simulink model "mbd_example_led"  (R2022b)
settings: Solver=FixedStepDiscrete  StartTime=0.0  StopTime=10.0  RelTol=1e-3  EnableMultiTasking=on
PostLoadFcn:
  | run([bdroot '_init']);
InitFcn:
  | checkModelFolder(true); % Optional
  | run([bdroot '_init']);
values from neighbouring files (symbols this model uses):
  T_s_LED1 = 1/LED1_Hz    (= 0.5)    [mbd_example_led_init.m]
  T_s_LED2 = 1/LED2_Hz    (= 1)    [mbd_example_led_init.m]
libraries: MbdLib_Digital x15, MbdLib_Timer x7, MbdLib_Sys x4, MbdLib_Required x1
(part 2 of 2)

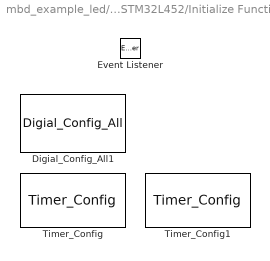
== system mbd_example_led/Variant Subsystem/STM32L452/Initialize Function ==
  Digial_Config_All1 : MbdLib_Digital/Digial_Config_All  Priority=30  Param_channels={ 'A', '0', 'off', '0 : input', '0 : low', '0 : none', '0 : none', '0 : low', '0 : low'; 'A', '1', 'off', '0 : input', '0 : low', '0 : none', '0 : none', '0 : low', '0 : low'; 'A', '2', 'off', '0 : input', '0 : low', '0 : none', '0 : none', '0 : low', '0 : low'; 'A', '3', 'off', '0 : input', '0 : low', '0 : none', '0 : none', '0 : low', '0 : low'; 'A', '4', 'off', '0 : input', '0 : low', '0 : none', '0 : none', '0 : low', '0 : low'; 'A', '5', 'off', '0 : input', '0 : low', '0 : none', '0 : none', '0 : low', '0 : low'; 'A', '6', 'off', '0 : input', '0 : low', '0 : none', '0 : none', '0 : low', '0 : low'; 'A', '7', 'off', '0 : input', '0 : low', '0 : none', '0 : none', '0 : low', '0 : low'; 'A', '8', 'off', '0 : input', '0 : low', '0 : none', '0 : none', '0 : low', '0 : low'; 'A', '9', 'off', '0 : input', '0 : low', '0 : none', '0 : none', '0 : low', '0 : low'; 'A', '10', 'off', '0 : input', '0 : low', '0 : none', '0 : none', '0 : low', '0 : low'; 'A', '11', 'off', '0 : input', '0 : low', '0 : none', '0 : none', '0 : low', '0 : low'; 'A', '12', 'off', '0 : input', '0 : low', '0 : none', '0 : none', '0 : low', '0 : low'; 'A', '13', 'off', '0 : input', '0 : low', '0 : none', '0 : none', '0 : low', '0 : low'; 'A', '14', 'off', '0 : input', '0 : low', '0 : none', '0 : none', '0 : low', '0 : low'; 'A', '15', 'off', '0 : input', '0 : low', '0 : none', '0 : none', '0 : low', '0 : low'; 'A', '16', 'off', '0 : input', '0 : low', '0 : none', '0 : none', '0 : low', '0 : low'; 'A', '17', 'off', '0 : input', '0 : low', '0 : none', '0 : none', '0 : low', '0 : low'; 'A', '18', 'off', '0 : input', '0 : low', '0 : none', '0 : none', '0 : low', '0 : low'; 'A', '19', 'off', '0 : input', '0 : low', '0 : none', '0 : none', '0 : low', '0 : low'; 'A', '20', 'off', '0 : input', '0 : low', '0 : none', '0 : none', '0 : low', '0 : low'; 'A', '21', 'off', '0 : input', '0 : low', '0 : none', '0 : none', '0 : low', '0 : low'; 'A', '22', 'off', '0 : input', '0 : low', '0 : none', '0 : none', '0 : low', '0 : low'; 'A', '23', 'off', '0 : input', '0 : low', '0 : none', '0 : none', '0 : low', '0 : low'; 'A', '24', 'off', '0 : input', '0 : low', '0 : none', '0 : none', '0 : low', '0 : low'; 'A', '25', 'off', '0 : input', '0 : low', '0 : none', '0 : none', '0 : low', '0 : low'; 'A', '26', 'off', '0 : input', '0 : low', '0 : none', '0 : none', '0 : low', '0 : low'; 'A', '27', 'off', '0 : input', '0 : low', '0 : none', '0 : none', '0 : low', '0 : low'; 'A', '28', 'off', '0 : input', '0 : low', '0 : none', '0 : none', '0 : low', '0 : low'; 'A', '29', 'off', '0 : input', '0 : low', '0 : none', '0 : none', '0 : low', '0 : low'; 'A', '30', 'off', '0 : input', '0 : low', '0 : none', '0 : none', '0 : low', '0 : low'; 'A', '31', 'off', '0 : input', '0 : low', '0 : none', '0 : none', '0 : low', '0 : low'; 'B', '0', 'off', '0 : input', '0 : low', '0 : none', '0 : none', '0 : low', '0 : low'; 'B', '1', 'off', '0 : input', '0 : low', '0 : none', '0 : none', '0 : low', '0 : low'; 'B', '2', 'off', '0 : input', '0 : low', '0 : none', '0 : none', '0 : low', '0 : low'; 'B', '3', 'off', '0 : input', '0 : low', '0 : none', '0 : none', '0 : low', '0 : low'; 'B', '4', 'off', '0 : input', '0 : low', '0 : none', '0 : none', '0 : low', '0 : low'; 'B', '5', 'off', '0 : input', '0 : low', '0 : none', '0 : none', '0 : low', '0 : low'; 'B', '6', 'off', '0 : input', '0 : low', '0 : none', '0 : none', '0 : low', '0 : low'; 'B', '7', 'off', '0 : input', '0 : low', '0 : none', '0 : none', '0 : low', '0 : low'; 'B', '8', 'off', '0 : input', '0 : low', '0 : none', '0 : none', '0 : low', '0 : low'; 'B', '9', 'off', '0 : input', '0 : low', '0 : none', '0 : none', '0 : low', '0 : low'; 'B', '10', 'off', '0 : input', '0 : low', '0 : none', '0 : none', '0 : low', '0 : low'; 'B', '11', 'off', '0 : input', '0 : low', '0 : none', '0 : none', '0 : low', '0 : low'; 'B', '12', 'off', '0 : input', '0 : low', '0 : none', '0 : none', '0 : low', '0 : low'; 'B', '13', 'off', '0 : input', '0 : low', '0 : none', '0 : none', '0 : low', '0 : low'; 'C', '0', 'off', '0 : input', '0 : low', '0 : none', '0 : none', '0 : low', '0 : low'; 'C', '1', 'off', '0 : input', '0 : low', '0 : none', '0 : none', '0 : low', '0 : low'; 'C', '2', 'off', '0 : input', '0 : low', '0 : none', '0 : none', '0 : low', '0 : low'; 'C', '3', 'off', '0 : input', '0 : low', '0 : none', '0 : none', '0 : low', '0 : low'; 'C', '4', 'off', '0 : input', '0 : low', '0 : none', '0 : none', '0 : low', '0 : low'; 'C', '5', 'off', '0 : input', '0 : low', '0 : none', '0 : none', '0 : low', '0 : low'; 'C', '6', 'off', '0 : input', '0 : low', '0 : none', '0 : none', '0 : low', '0 : low'; 'C', '7', 'off', '0 : input', '0 : low', '0 : none', '0 : none', '0 : low', '0 : low'; 'C', '8', 'off', '0 : input', '0 : low', '0 : none', '0 : none', '0 : low', '0 : low'; 'C', '9', 'off', '0 : input', '0 : low', '0 : none', '0 : none', '0 : low', '0 : low'; 'C', '10', 'on', '1 : output', '0 : low', '0 : none', '0 : none', '0 : low', '0 : low'; 'C', '11', 'off', '0 : input', '0 : low', '0 : none', '0 : none', '0 : low', '0 : low'; 'C', '12', 'off', '0 : input', '0 : low', '0 : none', '0 : none', '0 : low', '0 : low'; 'C', '13', 'on', '0 : input', '0 : low', '0 : none', '1 : pullup', '0 : low', '0 : low'; 'C', '14', 'off', '0 : input', '0 : low', '0 : none', '0 : none', '0 : low', '0 : low'; 'C', '15', 'off', '0 : input', '0 : low', '0 : none', '0 : none', '0 : low', '0 : low'; 'C', '16', 'off', '0 : input', '0 : low', '0 : none', '0 : none', '0 : low', '0 : low'; 'C', '17', 'off', '0 : input', '0 : low', '0 : none', '0 : none', '0 : low', '0 : low'; 'C', '18', 'off', '0 : input', '0 : low', '0 : none', '0 : none', '0 : low', '0 : low'; 'C', '19', 'off', '0 : input', '0 : low', '0 : none', '0 : none', '0 : low', '0 : low'; 'C', '20', 'off', '0 : input', '0 : low', '0 : none', '0 : none', '0 : low', '0 : low'; 'C', '21', 'off', '0 : input', '0 : low', '0 : none', '0 : none', '0 : low', '0 : low'; 'C', '22', 'off', '0 : input', '0 : low', '0 : none', '0 : none', '0 : low', '0 : low'; 'C', '23', 'off', '0 : input', '0 : low', '0 : none', '0 : none', '0 : low', '0 : low'; 'C', '24', 'off', '0 : input', '0 : low', '0 : none', '0 : none', '0 : low', '0 : low'; 'C', '25', 'off', '0 : input', '0 : low', '0 : none', '0 : none', '0 : low', '0 : low'; 'C', '26', 'off', '0 : input', '0 : low', '0 : none', '0 : none', '0 : low', '0 : low'; 'C', '27', 'off', '0 : input', '0 : low', '0 : none', '0 : none', '0 : low', '0 : low'; 'C', '28', 'off', '0 : input', '0 : low', '0 : none', '0 : none', '0 : low', '0 : low'; 'C', '29', 'off', '0 : input', '0 : low', '0 : none', '0 : none', '0 : low', '0 : low'; 'C', '30', 'off', '0 : input', '0 : low', '0 : none', '0 : none', '0 : low', '0 : low'; 'C', '31', 'off', '0 : input', '0 : low', '0 : none', '0 : none', '0 : low', '0 : low'; 'D', '0', 'off', '0 : input', '0 : low', '0 : none', '0 : none', '0 : low', '0 : low'; 'D', '1', 'off', '0 : input', '0 : low', '0 : none', '0 : none', '0 : low', '0 : low'; 'D', '2', 'off', '0 : input', '0 : low', '0 : none', '0 : none', '0 : low', '0 : low'; 'D', '3', 'off', '0 : input', '0 : low', '0 : none', '0 : none', '0 : low', '0 : low'; 'D', '4', 'off', '0 : input', '0 : low', '0 : none', '0 : none', '0 : low', '0 : low'; 'D', '5', 'off', '0 : input', '0 : low', '0 : none', '0 : none', '0 : low', '0 : low'; 'D', '6', 'off', '0 : input', '0 : low', '0 : none', '0 : none', '0 : low', '0 : low'; 'D', '7', 'off', '0 : input', '0 : low', '0 : none', '0 : none', '0 : low', '0 : low'; 'D', '8', 'off', '0 : input', '0 : low', '0 : none', '0 : none', '0 : low', '0 : low'; 'D', '9', 'off', '0 : input', '0 : low', '0 : none', '0 : none', '0 : low', '0 : low'; 'D', '10', 'off', '0 : input', '0 : low', '0 : none', '0 : none', '0 : low', '0 : low'; 'D', '11', 'off', '0 : input', '0 : low', '0 : none', '0 : none', '0 : low', '0 : low'; 'D', '12', 'off', '0 : input', '0 : low', '0 : none', '0 : none', '0 : low', '0 : low'; 'D', '13', 'off', '0 : input', '0 : low', '0 : none', '0 : none', '0 : low', '0 : low'; 'D', '14', 'off', '0 : input', '0 : low', '0 : none', '0 : none', '0 : low', '0 : low'; 'D', '15', 'off', '0 : input', '0 : low', '0 : none', '0 : none', '0 : low', '0 : low'; 'D', '16', 'off', '0 : input', '0 : low', '0 : none', '0 : none', '0 : low', '0 : low'; 'D', '17', 'off', '0 : input', '0 : low', '0 : none', '0 : none', '0 : low', '0 : low'; 'D', '18', 'off', '0 : input', '0 : low', '0 : none', '0 : none', '0 : low', '0 : low'; 'D', '19', 'off', '0 : input', '0 : low', '0 : none', '0 : none', '0 : low', '0 : low'; 'D', '20', 'off', '0 : input', '0 : low', '0 : none', '0 : none', '0 : low', '0 : low'; 'D', '21', 'off', '0 : input', '0 : low', '0 : none', '0 : none', '0 : low', '0 : low'; 'D', '22', 'off', '0 : input', '0 : low', '0 : none', '0 : none', '0 : low', '0 : low'; 'D', '23', 'off', '0 : input', '0 : low', '0 : none', '0 : none', '0 : low', '0 : low'; 'D', '24', 'off', '0 : input', '0 : low', '0 : none', '0 : none', '0 : low', '0 : low'; 'D', '25', 'off', '0 : input', '0 : low', '0 : none', '0 : none', '0 : low', '0 : low'; 'D', '26', 'off', '0 : input', '0 : low', '0 : none', '0 : none', '0 : low', '0 : low'; 'D', '27', 'off', '0 : input', '0 : low', '0 : none', '0 : none', '0 : low', '0 : low'; 'D', '28', 'off', '0 : input', '0 : low', '0 : none', '0 : none', '0 : low', '0 : low'; 'D', '29', 'off', '0 : input', '0 : low', '0 : none', '0 : none', '0 : low', '0 : low'; 'D', '30', 'off', '0 : input', '0 : low', '0 : none', '0 : none', '0 : low', '0 : low'; 'D', '31', 'off', '0 : input', '0 : low', '0 : none', '0 : none', '0 : low', '0 : low'; 'E', '0', 'off', '0 : input', '0 : low', '0 : none', '0 : none', '0 : low', '0 : low'; 'E', '1', 'off', '0 : input', '0 : low', '0 : none', '0 : none', '0 : low', '0 : low'; 'E', '2', 'off', '0 : input', '0 : low', '0 : none', '0 : none', '0 : low', '0 : low'; 'E', '3', 'off', '0 : input', '0 : low', '0 : none', '0 : none', '0 : low', '0 : low'; 'E', '4', 'off', '0 : input', '0 : low', '0 : none', '0 : none', '0 : low', '0 : low'; 'E', '5', 'off', '0 : input', '0 : low', '0 : none', '0 : none', '0 : low', '0 : low' }  Param_priority=30  Param_sampleTime=-1
      settings: AttributesFormatString=priority=%<priority>  SourceProductName=Peloton Interface Library
  Event Listener : EventListener  DisableCoverage=on  EventName=reset
  Timer_Config : MbdLib_Timer/Timer_Config  Priority=100  Param_update=1  Param_module=6  Param_step=0  Param_period=LED1_period_cycles  Param_divider=LED1_clock_divider  Param_step0=0  Param_clksrc0=0  Param_period0=LED1_period_cycles  Param_divider0=LED1_clock_divider  Param_step1=-1  Param_clksrc1=0  Param_period1=0  Param_divider1=0  Param_step2=-1  Param_clksrc2=0  Param_period2=0  Param_divider2=0  Param_priority=100  Param_sampleTime=-1
      settings: AttributesFormatString=priority=%<priority>  SourceProductName=Peloton Interface Library
  Timer_Config1 : MbdLib_Timer/Timer_Config  Priority=101  Param_update=1  Param_module=15  Param_step=1  Param_period=LED2_period_cycles  Param_divider=LED2_clock_divider  Param_step0=1  Param_clksrc0=0  Param_period0=LED2_period_cycles  Param_divider0=LED2_clock_divider  Param_step1=-1  Param_clksrc1=0  Param_period1=0  Param_divider1=0  Param_step2=-1  Param_clksrc2=0  Param_period2=0  Param_divider2=0  Param_priority=101  Param_sampleTime=-1
      settings: AttributesFormatString=priority=%<priority>  SourceProductName=Peloton Interface Library
